simulink model "tyden10_vili_starsi"  (R2020a)
settings: Solver=VariableStepAuto  StartTime=0.0  StopTime=10.0  RelTol=1e-3
values from neighbouring files (symbols this model uses):
  a1 = 2    [cv2.m]    (also in oprava5.m; setup.m; singular_polohy.m; test.m)
  a2 = 1.5    [cv2.m]    (also in oprava5.m; setup.m; singular_polohy.m; test.m)
  a3 = 0.5    [cv2.m]    (also in oprava5.m; setup.m; singular_polohy.m; test.m)
  s = surf(out.normdQ.time,fiss,dQ)    [sampleQnorm.m]
  T_1_0 = [cos(theta10), -sin(theta10), 0, a1*cos(theta10) ... (first row only)    [setup.m]
  T_2_1 = [cos(theta20), -sin(theta20), 0, a2*cos(theta20) ... (first row only)    [setup.m]
  T_3_2 = [cos(theta30), -sin(theta30), 0, a3*cos(theta30) ... (first row only)    [setup.m]
  X = A\b    [IGM.m]
undefined symbols (not defined in the file or in its folder): IGM, par, Y, Z
libraries: sm_lib x15, nesl_utility x7, simulink x5, fl_lib x1
settings Model: Creator=vilda  LastModifiedBy=Ja
settings DebuggingCC: SFMachineParentedDataDiag=error

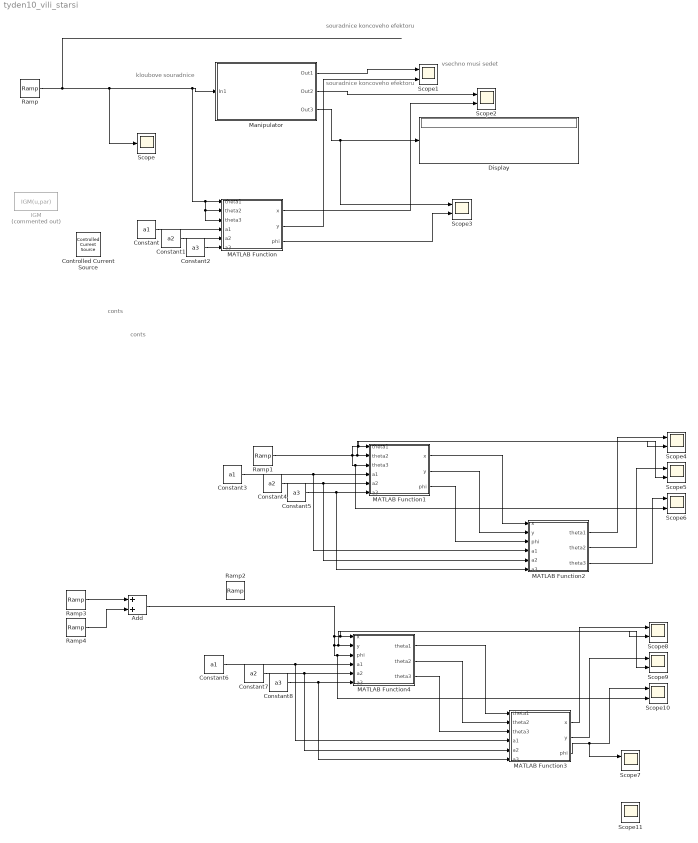
== system tyden10_vili_starsi ==
  note: conts
  note: conts
  note: vsechno musi sedet
  note: souradnice koncoveho efektoru
  note: kloubove souradnice
  note: souradnice koncoveho efektoru
  Add : Sum
  Constant : Constant  Value=a1
  Constant1 : Constant  Value=a2
  Constant2 : Constant  Value=a3
  Constant3 : Constant  Value=a1
  Constant4 : Constant  Value=a2
  Constant5 : Constant  Value=a3
  Constant6 : Constant  Value=a1
  Constant7 : Constant  Value=a2
  Constant8 : Constant  Value=a3
  Controlled Current Source : fl_lib/Electrical/Electrical Sources/Controlled Current Source
  Display : Display
  IGM : MATLABFcn  Commented=on  MATLABFcn=IGM(u,par)
  MATLAB Function : MATLAB Function  TreatAsAtomicUnit=on
  MATLAB Function1 : MATLAB Function  TreatAsAtomicUnit=on
  MATLAB Function2 : MATLAB Function  TreatAsAtomicUnit=on
  MATLAB Function3 : MATLAB Function  TreatAsAtomicUnit=on
  MATLAB Function4 : MATLAB Function  TreatAsAtomicUnit=on
  Manipulator : Subsystem
  Ramp{,1..3} (4 alike) : simulink/Sources/Ramp  slope=1  start=0  InitialOutput=0
  Ramp4 : simulink/Sources/Ramp  slope=-1  start=pi/2  InitialOutput=0
  Scope : Scope
  Scope{1..11} (11 alike) : Scope  NumInputPorts=2
  wires:
  Manipulator/1(Out1) -> Scope1/1
  Ramp/1 -> Scope/1, MATLAB Function/3(theta3), MATLAB Function/2(theta2), MATLAB Function/1(theta1), Manipulator/1(In1)
  Manipulator/2(Out2) -> Scope2/1
  Manipulator/3(Out3) -> Scope3/1, Display/1
  Constant2/1 -> MATLAB Function/6(a3)
  Constant1/1 -> MATLAB Function/5(a2)
  Constant/1 -> MATLAB Function/4(a1)
  MATLAB Function/1(x) -> Scope2/2
  MATLAB Function/2(y) -> Scope1/2
  MATLAB Function/3(phi) -> Scope3/2
  Constant5/1 -> MATLAB Function1/6(a3), MATLAB Function2/6(a3)
  Ramp1/1 -> Scope4/2, MATLAB Function1/1(theta1), Scope6/2, MATLAB Function1/3(theta3), Scope5/2, MATLAB Function1/2(theta2)
  Constant3/1 -> MATLAB Function1/4(a1), MATLAB Function2/4(a1)
  Constant4/1 -> MATLAB Function1/5(a2), MATLAB Function2/5(a2)
  MATLAB Function1/1(x) -> MATLAB Function2/1(x)
  MATLAB Function1/2(y) -> MATLAB Function2/2(y)
  MATLAB Function1/3(phi) -> MATLAB Function2/3(phi)
  MATLAB Function2/1(theta1) -> Scope4/1
  MATLAB Function2/2(theta2) -> Scope5/1
  MATLAB Function2/3(theta3) -> Scope6/1
  Add/1 -> MATLAB Function4/3(phi), Scope10/2, MATLAB Function4/2(y), Scope9/2, MATLAB Function4/1(x), Scope8/2
  MATLAB Function4/3(theta3) -> MATLAB Function3/3(theta3)
  MATLAB Function3/2(y) -> Scope9/1
  Constant6/1 -> MATLAB Function3/4(a1), MATLAB Function4/4(a1)
  Constant7/1 -> MATLAB Function3/5(a2), MATLAB Function4/5(a2)
  Constant8/1 -> MATLAB Function3/6(a3), MATLAB Function4/6(a3)
  MATLAB Function4/2(theta2) -> MATLAB Function3/2(theta2)
  MATLAB Function3/1(x) -> Scope8/1
  MATLAB Function4/1(theta1) -> MATLAB Function3/1(theta1)
  MATLAB Function3/3(phi) -> Scope7/1, Scope10/1
  Ramp3/1 -> Add/1
  Ramp4/1 -> Add/2
  ? -> Scope11/1

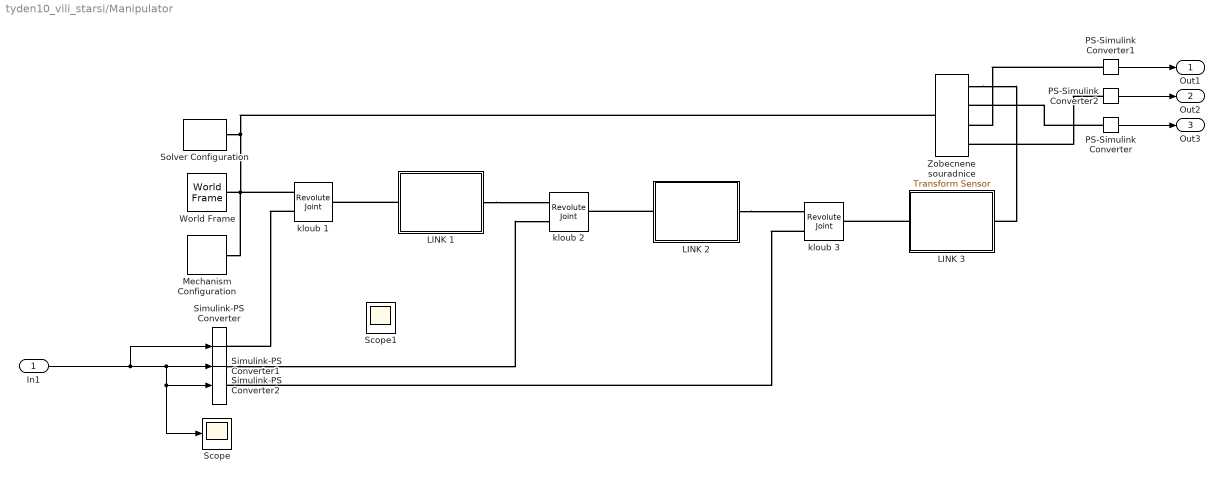
== system tyden10_vili_starsi/Manipulator ==
  In1 : Inport
  LINK 1 : Subsystem
  LINK 2 : Subsystem
  LINK 3 : Subsystem
  Mechanism Configuration : sm_lib/Utilities/Mechanism Configuration  UniformGravity=Constant  GravityVector=[0 0 -9.80665]  GravityUnits=m/s^2  LinearizationDelta=0.001
  PS-Simulink Converter : nesl_utility/PS-Simulink Converter  PhysicalDomain=network_engine_domain  SubClassName=ps_output  LeftPortType=input  RightPortType=output  PseudoPeriodic=off  Frequencies=[]  Unit=inherit  AffineConversion=off
      settings: SourceProductBaseCode=PW,SS
  PS-Simulink Converter1 : nesl_utility/PS-Simulink Converter  PhysicalDomain=network_engine_domain  SubClassName=ps_output  LeftPortType=input  RightPortType=output  PseudoPeriodic=off  Frequencies=[]  Unit=inherit  AffineConversion=off
      settings: SourceProductBaseCode=PW,SS
  PS-Simulink Converter2 : nesl_utility/PS-Simulink Converter  PhysicalDomain=network_engine_domain  SubClassName=ps_output  LeftPortType=input  RightPortType=output  PseudoPeriodic=off  Frequencies=[]  Unit=inherit  AffineConversion=off
      settings: SourceProductBaseCode=PW,SS
  Scope : Scope
  Scope1 : Scope
  Simulink-PS Converter : nesl_utility/Simulink-PS Converter  PhysicalDomain=network_engine_domain  SubClassName=ps_input  LeftPortType=input  RightPortType=output  PseudoPeriodic=off  Frequencies=[]  NoiseDistribution=none  NoiseParameters=[]  Unit=1  AffineConversion=off  FilteringAndDerivatives=filter  SimscapeFilterOrder=2  InputFilterTimeConstant=0.001  UdotUserProvided=0
      settings: SourceProductBaseCode=PW,SS
  Simulink-PS Converter1 : nesl_utility/Simulink-PS Converter  PhysicalDomain=network_engine_domain  SubClassName=ps_input  LeftPortType=input  RightPortType=output  PseudoPeriodic=off  Frequencies=[]  NoiseDistribution=none  NoiseParameters=[]  Unit=1  AffineConversion=off  FilteringAndDerivatives=filter  SimscapeFilterOrder=2  InputFilterTimeConstant=0.001  UdotUserProvided=0
      settings: SourceProductBaseCode=PW,SS
  Simulink-PS Converter2 : nesl_utility/Simulink-PS Converter  PhysicalDomain=network_engine_domain  SubClassName=ps_input  LeftPortType=input  RightPortType=output  PseudoPeriodic=off  Frequencies=[]  NoiseDistribution=none  NoiseParameters=[]  Unit=1  AffineConversion=off  FilteringAndDerivatives=filter  SimscapeFilterOrder=2  InputFilterTimeConstant=0.001  UdotUserProvided=0
      settings: SourceProductBaseCode=PW,SS
  Solver Configuration : nesl_utility/Solver Configuration  PhysicalDomain=network_engine_domain  SubClassName=solver  LeftPortType=input  RightPortType=generic  Tones=[]  Harmonics=[]  SimulateNoise=off  Profile=off  UseLocalSampling=off  EnableSwitchedLinearOptims=on  FrequencyDomain=off  UseCCode=off  RelTol=0.001  AbsTol=1e-06  MinStep=1e-09  ToWorkspace=off  RevertToSquareIcSolve=off  NumHomotopyIterations=100  PhasorMode=off  PhasorModeNumHarmonics=1  DoDC=off  ResidualTolerance=1e-09  UseLocalSolver=off  LocalSolverChoice=NE_BACKWARD_EULER_ADVANCER  LocalSolverSampleTime=0.001  DoFixedCost=off  MaxNonlinIter=3  MaxModeIter=2  LinearAlgebra=auto  EquationFormulation=NE_TIME_EF  DelaysMemoryBudget=1024  AutomaticFiltering=on  FilteringTimeConstant=0.001  PartitionStorageMethod=AS_NEEDED  PartitionMemoryBudget=1024  PartitionMethod=ROBUST
      settings: SourceProductBaseCode=PW,SS
  World Frame : sm_lib/Frames and Transforms/World Frame
  Zobecnene souradnice : sm_lib/Frames and Transforms/Transform Sensor  MeasurementFrame=World  SenseAngle=on  SenseAxis=off  SenseAngle1=off  SenseAngle2=off  SenseAngle3=off  SenseQ=off  SenseR=off  SenseOmegaX=off  SenseOmegaY=off  SenseOmegaZ=off  SenseOmega1=off  SenseOmega2=off  SenseOmega3=off  SenseQDot=off  SenseRDot=off  SenseAlphaX=off  SenseAlphaY=off  SenseAlphaZ=off  SenseAlpha1=off  SenseAlpha2=off  SenseAlpha3=off  SenseQDDot=off  SenseRDDot=off  SenseX=on  SenseY=on  SenseZ=off  SenseRad=off  SenseAzim=off  SenseDist=off  SenseInc=off  SenseXDot=off  SenseYDot=off  SenseZDot=off  SenseRadDot=off  SenseAzimDot=off  SenseDistDot=off  SenseIncDot=off  SenseXDDot=off  SenseYDDot=off  SenseZDDot=off  SenseRadDDot=off  SenseAzimDDot=off  SenseDistDDot=off  SenseIncDDot=off
  kloub 1 : sm_lib/Joints/Revolute Joint  JointMode=Normal  SenseConstraintForce=off  SenseConstraintForceX=off  SenseConstraintForceY=off  SenseConstraintForceZ=off  SenseConstraintTorque=off  SenseConstraintTorqueX=off  SenseConstraintTorqueY=off  SenseConstraintTorqueZ=off  SenseTotalForce=off  SenseTotalForceX=off  SenseTotalForceY=off  SenseTotalForceZ=off  SenseTotalTorque=off  SenseTotalTorqueX=off  SenseTotalTorqueY=off  SenseTotalTorqueZ=off  CompositeWrenchDir=FollowerOnBase  CompositeWrenchFrame=BaseFrame  EquilibriumPosition=0  EquilibriumPositionUnits=deg  SpringStiffness=0  SpringStiffnessUnits=N*m/deg  DampingCoefficient=0  DampingCoefficientUnits=N*m/(deg/s)  TorqueActuationMode=ComputedTorque  MotionActuationMode=InputMotion  SensePosition=off  SenseVelocity=off  SenseAcceleration=off  SenseTorqueForce=off  SenseLowerLimitTorqueForce=off  SenseUpperLimitTorqueForce=off  LowerLimitSpecify=off  LowerLimitBound=-90  LowerLimitBoundUnits=deg  LowerLimitStiffness=1e4  LowerLimitStiffnessUnits=N*m/deg  LowerLimitDamping=10  LowerLimitDampingUnits=N*m/(deg/s)  LowerLimitTransitionRegionWidth=0.1  LowerLimitTransitionRegionWidthUnits=deg  UpperLimitSpecify=off  UpperLimitBound=90  UpperLimitBoundUnits=deg  UpperLimitStiffness=1e4  UpperLimitStiffnessUnits=N*m/deg  UpperLimitDamping=10  UpperLimitDampingUnits=N*m/(deg/s)  UpperLimitTransitionRegionWidth=0.1  UpperLimitTransitionRegionWidthUnits=deg  PositionTargetSpecify=off  PositionTargetPriority=High  PositionTargetValue=0  PositionTargetValueUnits=deg  VelocityTargetSpecify=off  VelocityTargetPriority=High  VelocityTargetValue=0  VelocityTargetValueUnits=deg/s
  kloub 2 : sm_lib/Joints/Revolute Joint  JointMode=Normal  SenseConstraintForce=off  SenseConstraintForceX=off  SenseConstraintForceY=off  SenseConstraintForceZ=off  SenseConstraintTorque=off  SenseConstraintTorqueX=off  SenseConstraintTorqueY=off  SenseConstraintTorqueZ=off  SenseTotalForce=off  SenseTotalForceX=off  SenseTotalForceY=off  SenseTotalForceZ=off  SenseTotalTorque=off  SenseTotalTorqueX=off  SenseTotalTorqueY=off  SenseTotalTorqueZ=off  CompositeWrenchDir=FollowerOnBase  CompositeWrenchFrame=BaseFrame  EquilibriumPosition=0  EquilibriumPositionUnits=deg  SpringStiffness=0  SpringStiffnessUnits=N*m/deg  DampingCoefficient=0  DampingCoefficientUnits=N*m/(deg/s)  TorqueActuationMode=ComputedTorque  MotionActuationMode=InputMotion  SensePosition=off  SenseVelocity=off  SenseAcceleration=off  SenseTorqueForce=off  SenseLowerLimitTorqueForce=off  SenseUpperLimitTorqueForce=off  LowerLimitSpecify=off  LowerLimitBound=-90  LowerLimitBoundUnits=deg  LowerLimitStiffness=1e4  LowerLimitStiffnessUnits=N*m/deg  LowerLimitDamping=10  LowerLimitDampingUnits=N*m/(deg/s)  LowerLimitTransitionRegionWidth=0.1  LowerLimitTransitionRegionWidthUnits=deg  UpperLimitSpecify=off  UpperLimitBound=90  UpperLimitBoundUnits=deg  UpperLimitStiffness=1e4  UpperLimitStiffnessUnits=N*m/deg  UpperLimitDamping=10  UpperLimitDampingUnits=N*m/(deg/s)  UpperLimitTransitionRegionWidth=0.1  UpperLimitTransitionRegionWidthUnits=deg  PositionTargetSpecify=off  PositionTargetPriority=High  PositionTargetValue=0  PositionTargetValueUnits=deg  VelocityTargetSpecify=off  VelocityTargetPriority=High  VelocityTargetValue=0  VelocityTargetValueUnits=deg/s
  kloub 3 : sm_lib/Joints/Revolute Joint  JointMode=Normal  SenseConstraintForce=off  SenseConstraintForceX=off  SenseConstraintForceY=off  SenseConstraintForceZ=off  SenseConstraintTorque=off  SenseConstraintTorqueX=off  SenseConstraintTorqueY=off  SenseConstraintTorqueZ=off  SenseTotalForce=off  SenseTotalForceX=off  SenseTotalForceY=off  SenseTotalForceZ=off  SenseTotalTorque=off  SenseTotalTorqueX=off  SenseTotalTorqueY=off  SenseTotalTorqueZ=off  CompositeWrenchDir=FollowerOnBase  CompositeWrenchFrame=BaseFrame  EquilibriumPosition=0  EquilibriumPositionUnits=deg  SpringStiffness=0  SpringStiffnessUnits=N*m/deg  DampingCoefficient=0  DampingCoefficientUnits=N*m/(deg/s)  TorqueActuationMode=ComputedTorque  MotionActuationMode=InputMotion  SensePosition=off  SenseVelocity=off  SenseAcceleration=off  SenseTorqueForce=off  SenseLowerLimitTorqueForce=off  SenseUpperLimitTorqueForce=off  LowerLimitSpecify=off  LowerLimitBound=-90  LowerLimitBoundUnits=deg  LowerLimitStiffness=1e4  LowerLimitStiffnessUnits=N*m/deg  LowerLimitDamping=10  LowerLimitDampingUnits=N*m/(deg/s)  LowerLimitTransitionRegionWidth=0.1  LowerLimitTransitionRegionWidthUnits=deg  UpperLimitSpecify=off  UpperLimitBound=90  UpperLimitBoundUnits=deg  UpperLimitStiffness=1e4  UpperLimitStiffnessUnits=N*m/deg  UpperLimitDamping=10  UpperLimitDampingUnits=N*m/(deg/s)  UpperLimitTransitionRegionWidth=0.1  UpperLimitTransitionRegionWidthUnits=deg  PositionTargetSpecify=off  PositionTargetPriority=High  PositionTargetValue=0  PositionTargetValueUnits=deg  VelocityTargetSpecify=off  VelocityTargetPriority=High  VelocityTargetValue=0  VelocityTargetValueUnits=deg/s
  Out1 : Outport
  Out2 : Outport  Port=2
  Out3 : Outport  Port=3
  wires:
  PS-Simulink Converter1/1 -> Out1/1
  In1/1 -> Scope/1, Simulink-PS Converter2/1, Simulink-PS Converter1/1, Simulink-PS Converter/1
  PS-Simulink Converter2/1 -> Out2/1
  PS-Simulink Converter/1 -> Out3/1
  ? -> Scope1/1
  connections:
  LINK 3/LConn1 -- kloub 3/RConn1
  kloub 1/LConn2 -- Simulink-PS Converter/RConn1
  LINK 2/RConn1 -- kloub 3/LConn1
  LINK 1/RConn1 -- kloub 2/LConn1
  Solver Configuration/RConn1 -- Zobecnene souradnice/LConn1 -- Mechanism Configuration/RConn1 -- kloub 1/LConn1 -- World Frame/RConn1
  Simulink-PS Converter1/RConn1 -- kloub 2/LConn2
  Zobecnene souradnice/RConn1 -- LINK 3/RConn1
  LINK 2/LConn1 -- kloub 2/RConn1
  kloub 3/LConn2 -- Simulink-PS Converter2/RConn1
  LINK 1/LConn1 -- kloub 1/RConn1
  PS-Simulink Converter/LConn1 -- Zobecnene souradnice/RConn2
  PS-Simulink Converter2/LConn1 -- Zobecnene souradnice/RConn4
  PS-Simulink Converter1/LConn1 -- Zobecnene souradnice/RConn3

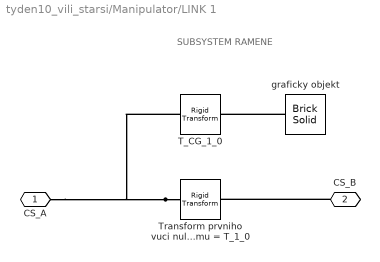
== system tyden10_vili_starsi/Manipulator/LINK 1 ==
  note: SUBSYSTEM RAMENE
  T_CG_1_0 : sm_lib/Frames and Transforms/Rigid Transform  TranslationMethod=Cartesian  TranslationStandardOffset=0  TranslationLengthUnit=m  TranslationStandardAxis=+Z  TranslationCartesianOffset=T_1_0(1:3,4)/2  TranslationROffset=0  TranslationROffsetUnits=m  TranslationZOffset=0  TranslationZOffsetUnits=m  TranslationThetaOffset=0  TranslationThetaOffsetUnits=deg  RotationMethod=RotationMatrix  RotationAngleUnits=deg  RotationStandardAxis=+Z  RotationAngle=0.0  RotationArbitraryAxis=[0 0 1]  FollAlignAxisA=+X  BaseAlignAxisA=+Y  FollAlignAxisB=+Y  BaseAlignAxisB=+Z  RotationSequenceAxes=FollowerAxes  RotationSequence=XYX  RotationSequenceAngles=[0 0 0]  RotationSequenceAnglesUnits=deg  RotationMatrix=T_1_0(1:3,1:3)
  Transform prvniho vuci nultymu = T_1_0 : sm_lib/Frames and Transforms/Rigid Transform  TranslationMethod=Cartesian  TranslationStandardOffset=0  TranslationLengthUnit=m  TranslationStandardAxis=+Z  TranslationCartesianOffset=T_1_0(1:3,4)  TranslationROffset=0  TranslationROffsetUnits=m  TranslationZOffset=0  TranslationZOffsetUnits=m  TranslationThetaOffset=0  TranslationThetaOffsetUnits=deg  RotationMethod=RotationMatrix  RotationAngleUnits=deg  RotationStandardAxis=+Z  RotationAngle=0.0  RotationArbitraryAxis=[0 0 1]  FollAlignAxisA=+X  BaseAlignAxisA=+Y  FollAlignAxisB=+Y  BaseAlignAxisB=+Z  RotationSequenceAxes=FollowerAxes  RotationSequence=XYX  RotationSequenceAngles=[0 0 0]  RotationSequenceAnglesUnits=deg  RotationMatrix=T_1_0(1:3,1:3)
  graficky objekt : sm_lib/Body Elements/Brick Solid  GraphicAmbientColor=[0.15 0.15 0.15 1.0]  BasedOnType=Density  BrickDimensions=[a1 0.05 0.05]  BrickDimensionUnits=m  CenterOfMass=[0 0 0]  CenterOfMassUnits=m  GraphicDiffuseColor=[0.5 0.5 0.5]  Density=1000  DensityUnits=kg/m^3  DoExposeReferenceFrame=on  GraphicEmissiveColor=[0.0 0.0 0.0 1.0]  ExportEntireGeometry=off  SerializedFrames=<Frames/>  MarkerShape=Sphere  MarkerSize=10  GraphicType=FromGeometry  InertiaType=CalculateFromGeometry  Mass=1  MassUnits=kg  MomentsOfInertia=[1 1 1]  MomentsOfInertiaUnits=kg*m^2  GraphicOpacity=1.0  ProductsOfInertia=[0 0 0]  ProductsOfInertiaUnits=kg*m^2  GraphicShininess=75  GraphicSpecularColor=[0.5 0.5 0.5 1.0]  GraphicVisPropType=SimpleVisualProperties
  CS_A : PMIOPort  Side=Left
  CS_B : PMIOPort  Port=2  Side=Right
  connections:
  Transform prvniho vuci nultymu = T_1_0/LConn1 -- CS_A/RConn1 -- T_CG_1_0/LConn1
  CS_B/RConn1 -- Transform prvniho vuci nultymu = T_1_0/RConn1
  graficky objekt/RConn1 -- T_CG_1_0/RConn1

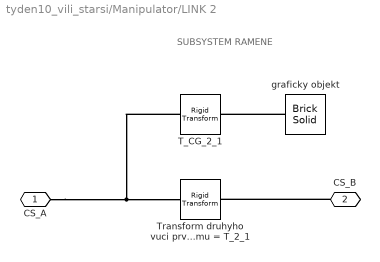
== system tyden10_vili_starsi/Manipulator/LINK 2 ==
  note: SUBSYSTEM RAMENE
  T_CG_2_1 : sm_lib/Frames and Transforms/Rigid Transform  TranslationMethod=Cartesian  TranslationStandardOffset=0  TranslationLengthUnit=m  TranslationStandardAxis=+Z  TranslationCartesianOffset=T_2_1(1:3,4)/2  TranslationROffset=0  TranslationROffsetUnits=m  TranslationZOffset=0  TranslationZOffsetUnits=m  TranslationThetaOffset=0  TranslationThetaOffsetUnits=deg  RotationMethod=RotationMatrix  RotationAngleUnits=deg  RotationStandardAxis=+Z  RotationAngle=0.0  RotationArbitraryAxis=[0 0 1]  FollAlignAxisA=+X  BaseAlignAxisA=+Y  FollAlignAxisB=+Y  BaseAlignAxisB=+Z  RotationSequenceAxes=FollowerAxes  RotationSequence=XYX  RotationSequenceAngles=[0 0 0]  RotationSequenceAnglesUnits=deg  RotationMatrix=T_2_1(1:3,1:3)
  Transform druhyho vuci prvnimu = T_2_1 : sm_lib/Frames and Transforms/Rigid Transform  TranslationMethod=Cartesian  TranslationStandardOffset=0  TranslationLengthUnit=m  TranslationStandardAxis=+Z  TranslationCartesianOffset=T_2_1(1:3,4)  TranslationROffset=0  TranslationROffsetUnits=m  TranslationZOffset=0  TranslationZOffsetUnits=m  TranslationThetaOffset=0  TranslationThetaOffsetUnits=deg  RotationMethod=RotationMatrix  RotationAngleUnits=deg  RotationStandardAxis=+Z  RotationAngle=0.0  RotationArbitraryAxis=[0 0 1]  FollAlignAxisA=+X  BaseAlignAxisA=+Y  FollAlignAxisB=+Y  BaseAlignAxisB=+Z  RotationSequenceAxes=FollowerAxes  RotationSequence=XYX  RotationSequenceAngles=[0 0 0]  RotationSequenceAnglesUnits=deg  RotationMatrix=T_2_1(1:3,1:3)
  graficky objekt : sm_lib/Body Elements/Brick Solid  GraphicAmbientColor=[0.15 0.15 0.15 1.0]  BasedOnType=Density  BrickDimensions=[a2 0.05 0.05]  BrickDimensionUnits=m  CenterOfMass=[0 0 0]  CenterOfMassUnits=m  GraphicDiffuseColor=[0.5 0.5 0.5]  Density=1000  DensityUnits=kg/m^3  DoExposeReferenceFrame=on  GraphicEmissiveColor=[0.0 0.0 0.0 1.0]  ExportEntireGeometry=off  SerializedFrames=<Frames/>  MarkerShape=Sphere  MarkerSize=10  GraphicType=FromGeometry  InertiaType=CalculateFromGeometry  Mass=1  MassUnits=kg  MomentsOfInertia=[1 1 1]  MomentsOfInertiaUnits=kg*m^2  GraphicOpacity=1.0  ProductsOfInertia=[0 0 0]  ProductsOfInertiaUnits=kg*m^2  GraphicShininess=75  GraphicSpecularColor=[0.5 0.5 0.5 1.0]  GraphicVisPropType=SimpleVisualProperties
  CS_A : PMIOPort  Side=Left
  CS_B : PMIOPort  Port=2  Side=Right
  connections:
  T_CG_2_1/LConn1 -- Transform druhyho vuci prvnimu = T_2_1/LConn1 -- CS_A/RConn1
  CS_B/RConn1 -- Transform druhyho vuci prvnimu = T_2_1/RConn1
  graficky objekt/RConn1 -- T_CG_2_1/RConn1

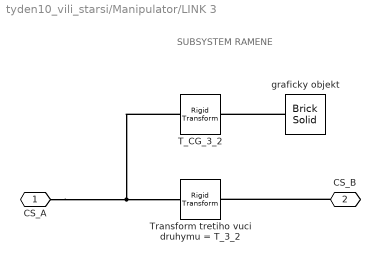
== system tyden10_vili_starsi/Manipulator/LINK 3 ==
  note: SUBSYSTEM RAMENE
  T_CG_3_2 : sm_lib/Frames and Transforms/Rigid Transform  TranslationMethod=Cartesian  TranslationStandardOffset=0  TranslationLengthUnit=m  TranslationStandardAxis=+Z  TranslationCartesianOffset=T_3_2(1:3,4)/2  TranslationROffset=0  TranslationROffsetUnits=m  TranslationZOffset=0  TranslationZOffsetUnits=m  TranslationThetaOffset=0  TranslationThetaOffsetUnits=deg  RotationMethod=RotationMatrix  RotationAngleUnits=deg  RotationStandardAxis=+Z  RotationAngle=0.0  RotationArbitraryAxis=[0 0 1]  FollAlignAxisA=+X  BaseAlignAxisA=+Y  FollAlignAxisB=+Y  BaseAlignAxisB=+Z  RotationSequenceAxes=FollowerAxes  RotationSequence=XYX  RotationSequenceAngles=[0 0 0]  RotationSequenceAnglesUnits=deg  RotationMatrix=T_3_2(1:3,1:3)
  Transform tretiho vuci druhymu = T_3_2 : sm_lib/Frames and Transforms/Rigid Transform  TranslationMethod=Cartesian  TranslationStandardOffset=0  TranslationLengthUnit=m  TranslationStandardAxis=+Z  TranslationCartesianOffset=T_3_2(1:3,4)  TranslationROffset=0  TranslationROffsetUnits=m  TranslationZOffset=0  TranslationZOffsetUnits=m  TranslationThetaOffset=0  TranslationThetaOffsetUnits=deg  RotationMethod=RotationMatrix  RotationAngleUnits=deg  RotationStandardAxis=+Z  RotationAngle=0.0  RotationArbitraryAxis=[0 0 1]  FollAlignAxisA=+X  BaseAlignAxisA=+Y  FollAlignAxisB=+Y  BaseAlignAxisB=+Z  RotationSequenceAxes=FollowerAxes  RotationSequence=XYX  RotationSequenceAngles=[0 0 0]  RotationSequenceAnglesUnits=deg  RotationMatrix=T_3_2(1:3,1:3)
  graficky objekt : sm_lib/Body Elements/Brick Solid  GraphicAmbientColor=[0.15 0.15 0.15 1.0]  BasedOnType=Density  BrickDimensions=[a3 0.05 0.05]  BrickDimensionUnits=m  CenterOfMass=[0 0 0]  CenterOfMassUnits=m  GraphicDiffuseColor=[0.5 0.5 0.5]  Density=1000  DensityUnits=kg/m^3  DoExposeReferenceFrame=on  GraphicEmissiveColor=[0.0 0.0 0.0 1.0]  ExportEntireGeometry=off  SerializedFrames=<Frames/>  MarkerShape=Sphere  MarkerSize=10  GraphicType=FromGeometry  InertiaType=CalculateFromGeometry  Mass=1  MassUnits=kg  MomentsOfInertia=[1 1 1]  MomentsOfInertiaUnits=kg*m^2  GraphicOpacity=1.0  ProductsOfInertia=[0 0 0]  ProductsOfInertiaUnits=kg*m^2  GraphicShininess=75  GraphicSpecularColor=[0.5 0.5 0.5 1.0]  GraphicVisPropType=SimpleVisualProperties
  CS_A : PMIOPort  Side=Left
  CS_B : PMIOPort  Port=2  Side=Right
  connections:
  T_CG_3_2/LConn1 -- Transform tretiho vuci druhymu = T_3_2/LConn1 -- CS_A/RConn1
  CS_B/RConn1 -- Transform tretiho vuci druhymu = T_3_2/RConn1
  graficky objekt/RConn1 -- T_CG_3_2/RConn1

== matlab function tyden10_vili_starsi/MATLAB Function1 ==
  data: x output; theta1 input; y output; theta2 input; theta3 input; a1 input; a2 input; a3 input; phi output
function [x,y,phi] = DGM(theta1, theta2, theta3,a1,a2,a3)
   x = a3*cos(theta1+theta2+theta3) + a2*cos(theta1+theta2) + a1*cos(theta1);
   y = a3*sin(theta1+theta2+theta3) + a2*sin(theta1+theta2) + a1*sin(theta1);
   phi = atan2(sin(theta1+theta2+theta3),cos(theta1+theta2+theta3));
end

== matlab function tyden10_vili_starsi/MATLAB Function ==
  data: x output; theta1 input; y output; theta2 input; theta3 input; a1 input; a2 input; a3 input; phi output
function [x,y,phi] = DGM(theta1, theta2, theta3,a1,a2,a3)
   x = a3*cos(theta1+theta2+theta3) + a2*cos(theta1+theta2) + a1*cos(theta1);
   y = a3*sin(theta1+theta2+theta3) + a2*sin(theta1+theta2) + a1*sin(theta1);
   phi = atan2(sin(theta1+theta2+theta3),cos(theta1+theta2+theta3));
end

== matlab function tyden10_vili_starsi/MATLAB Function2 ==
  data: theta1 output size=1; x input; theta2 output size=1; y input; phi input; a1 input; a2 input; a3 input; theta3 output size=1
function [theta1, theta2, theta3] = IGM( x, y, phi, a1, a2, a3)
    cosQ2 = ((x - a3 *cos(phi))^2 + (y - a3 * sin(phi))^2 - a2^2 - a1^2)/(2*a1*a2);
    sinQ2 = - abs( sqrt(1 - cosQ2)); % 2 reseni, vybereme -
    
    theta2 = atan2(sinQ2, cosQ2); % Q2
    A = [-a2 * sinQ2, a2*cosQ2 + a1;
         a2 * cosQ2 + a1, -a2*sinQ2];
    b = [x - a3 * cos(phi); y - a3 * sin(phi)];
    
    X = A\b;
%     sin(theta1) = X(1);
%     cos(theta1) = X(2);
    
    theta1 = atan2(X(1),X(2)); % Q1
    
    theta3 = phi - theta2 - theta1; % Q3
end

== matlab function tyden10_vili_starsi/MATLAB Function3 ==
  data: x output; theta1 input; y output; theta2 input; theta3 input; a1 input; a2 input; a3 input; phi output
function [x,y,phi] = DGM(theta1, theta2, theta3,a1,a2,a3)
   x = a3*cos(theta1+theta2+theta3) + a2*cos(theta1+theta2) + a1*cos(theta1);
   y = a3*sin(theta1+theta2+theta3) + a2*sin(theta1+theta2) + a1*sin(theta1);
   phi = atan2(sin(theta1+theta2+theta3),cos(theta1+theta2+theta3));
%    phi2 = theta1+theta2+theta3
end

== matlab function tyden10_vili_starsi/MATLAB Function4 ==
  data: theta1 output size=1; x input; theta2 output size=1; y input; phi input; a1 input; a2 input; a3 input; theta3 output size=1
function [theta1, theta2, theta3] = IGM( x, y, phi, a1, a2, a3)
    cosQ2 = ((x - a3 *cos(phi))^2 + (y - a3 * sin(phi))^2 - a2^2 - a1^2)/(2*a1*a2);
    sinQ2 = - abs(sqrt(1 - cosQ2)); % 2 reseni, vybereme -
    
    theta2 = atan2(sinQ2, cosQ2); % Q2
    A = [-a2 * sinQ2, a2*cosQ2 + a1;
         a2 * cosQ2 + a1, a2*sinQ2];
    b = [x - a3 * cos(phi); y - a3 * sin(phi)];
    
    X = A\b;
%     sin(theta1) = X(1);
%     cos(theta1) = X(2);
    
    theta1 = atan2(X(1),X(2)); % Q1
    
    theta3 = phi - theta2 - theta1; % Q3
end
